simulink model "HyEQ_Optimized"  (Simulink 7.7)
settings: Solver=ode45  StartTime=0.0  StopTime=T  MaxStep=MaxStep  RelTol=RelTol
undefined symbols (not defined in the file or in its folder): J, rule, T, x0
libraries: simulink x6
settings Model: Creator=pablonanez  LastModifiedBy=pablonanez
settings SFSimCC: SimParseCustomCode=off

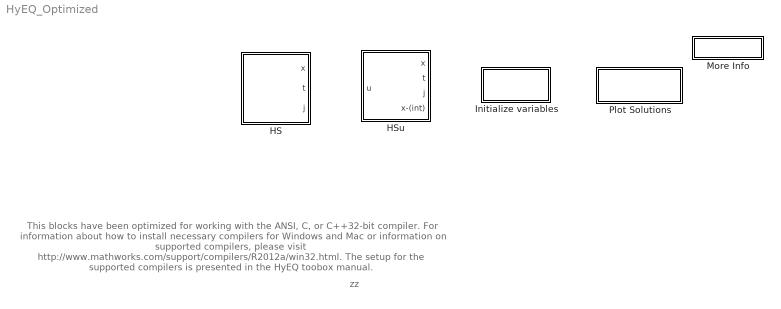
== system HyEQ_Optimized ==
  note: zz
  note: This blocks have been optimized for working with the ANSI, C, or C++32-bit compiler.
      |
      | For information about how to install necessary compilers for Windows and Mac or
      | information on supported compilers, please visit
      | http://www.mathworks.com/support/compilers/R2012a/win32.html.
      |
      | The setup for the supported compilers is presented in the HyEQ toobox manual.
  HS : Subsystem  LoadFcn=set_param(gcb,'LinkStatus','none')
      settings: CopyFcn=|
      | set_param(gcb,'LinkStatus','none'),
      | set_param(gcs, 'MaxStep', 'MaxStep', 'RelTol','RelTol','Stop time', 'T')
      mask Display:
      | image(imread('Hcal.jpg'))
      | %plot([5 20 20 5 5],[5 5 20 20 5])
      | %text(8,13,'HyEq_mdl')
      | port_label('output', 1, 'x')
      | port_label('output', 2, 't')
      | port_label('output', 3, 'j')
  HSu : Subsystem  LoadFcn=set_param(gcb,'LinkStatus','none')
      settings: CopyFcn=|
      | set_param(gcb,'LinkStatus','none'),
      | set_param(gcs, 'MaxStep', 'MaxStep', 'RelTol', 'RelTol','Stop time', 'T')
      mask Display:
      | image(imread('Hcal.jpg'))
      | %plot([5 20 20 5 5],[5 5 20 20 5])
      | %text(8,13,'HyEq_mdl')
      | port_label('output', 1, 'x')
      | port_label('output', 2, 't')
      | port_label('output', 3, 'j')
      | port_label('output', 4, 'x-(int)')
      | port_label('input', 1, 'u')
  Initialize variables : Subsystem  Priority=-10
      settings: OpenFcn=|
      | try
      |      clearvars -except inifile pathfile_in pathfile_pos posfile
      |      cd(pathfile_in);
      |      eval(inifile);
      | catch
      |      [inifile,pathfile_in] = getInitializationfile;
      |      cd(pathfile_in);
      |      inifile = strrep(inifile,'.m','');
      |      eval(inifile);
      | end
      mask Display: disp('Double Click\n to Initialize')
  More Info : Subsystem
      settings: OpenFcn=helpview 'HyEQ_Toolbox_v201.html'
      mask Display: disp('More Info')
  Plot Solutions : Subsystem
      settings: OpenFcn=|
      | try
      |      cd(pathfile_pos);
      |      eval(posfile);
      | catch
      |      [posfile,pathfile_pos] = getInitializationfile;
      |      cd(pathfile_pos);
      |      posfile = strrep(posfile,'.m','');
      |      eval(posfile);
      | end
      mask Display: disp('Double Click to\n Plot Solutions')

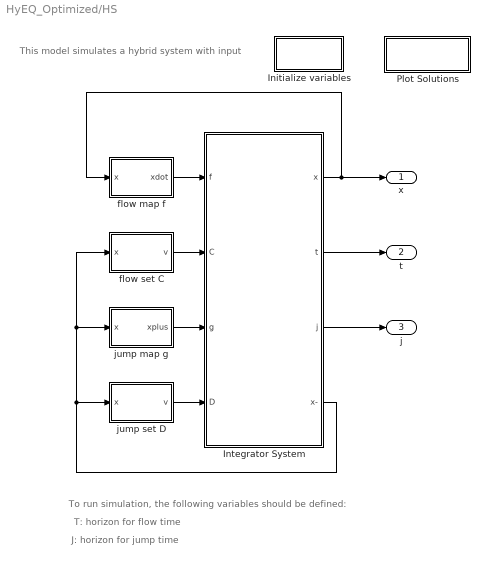
== system HyEQ_Optimized/HS ==
  note: This model simulates a hybrid system with input
  note: To run simulation, the following variables should be defined:
  note: T: horizon for flow time
  note: J: horizon for jump time
  Initialize variables : Subsystem  Priority=-10
      settings: OpenFcn=|
      | try
      |      clearvars -except inifile pathfile_in pathfile_pos posfile
      |      cd(pathfile_in);
      |      eval(inifile);
      | catch
      |      [inifile,pathfile_in] = getInitializationfile;
      |      cd(pathfile_in);
      |      inifile = strrep(inifile,'.m','');
      |      eval(inifile);
      | end
      mask Display: disp('Double Click\n to Initialize')
  Integrator System : Subsystem  Priority=2  mask(Hybrid Integrator){T=T, J=J, x0=x0}
      mask prompts: T "Flow Horizon"; J "Jump Horizon"; x0 "Initial Condition"
      mask help:
      | This block integrates the state of the hybrid system defined by the flow map f (first input), the flow set C (second input), the jump map g (third input) and the jump set D (fourth input).
      | Starting from the initial condition x0 (last mask parameter), the system's state x evolves continuously within the set C, according to f(x,u), but is also subject to jumps within D, according to g(x,u).
      | The block also stops the simulation when the time t is greater than the flow horizon T (first mask parameter), or when the number of jumps j is greater than the jump horizon J (second mask parameter).
      | The outputs of the blocks are respectively x(t), t, j, x(t-).
      mask Help:
      | This block integrates the state of the hybrid system defined by the flow map f (first input), the flow set C (second input), the jump map g (third input) and the jump set D (fourth input).
      | <br>
      | Starting from the initial condition x0 (last mask parameter), the system's state x evolves continuously within the set C, according to f(x,u), but is also subject to jumps within D, according to g(x,u).
      | <br>
      | The block also stops the simulation when the time t is greater than the flow horizon T (first mask parameter), or when the number of jumps j is greater than the jump horizon J (second mask parameter).
      | <br>
      | The outputs of the blocks are respectively x(t), t, j, x(t-).
      | <br>
      | You can right click on the block and "Look under mask" to see what's inside the block.
      | Finally, refer to the manual (HybridSimulator_vXX.pdf) for more detailed information on how this hybrid simulator works.
  Plot Solutions : Subsystem
      settings: OpenFcn=|
      | try
      |      cd(pathfile_pos);
      |      eval(posfile);
      | catch
      |      [posfile,pathfile_pos] = getInitializationfile;
      |      cd(pathfile_pos);
      |      posfile = strrep(posfile,'.m','');
      |      eval(posfile);
      | end
      mask Display: disp('Double Click to\n Plot Solutions')
  flow map f : Stateflow chart  TreatAsAtomicUnit=on
  flow set C : Stateflow chart  TreatAsAtomicUnit=on
  jump map g : Stateflow chart  Priority=2  TreatAsAtomicUnit=on
  jump set D : Stateflow chart  TreatAsAtomicUnit=on
  x : Outport
  t : Outport  Port=2
  j : Outport  Port=3
  wires:
  flow map f/1(xdot) -> Integrator System/1(f)
  Integrator System/4(x-) -> jump map g/1(x), flow set C/1(x), jump set D/1(x)
  Integrator System/1(x) -> flow map f/1(x), x/1
  flow set C/1(v) -> Integrator System/2(C)
  Integrator System/2(t) -> t/1
  Integrator System/3(j) -> j/1
  jump set D/1(v) -> Integrator System/4(D)
  jump map g/1(xplus) -> Integrator System/3(g)

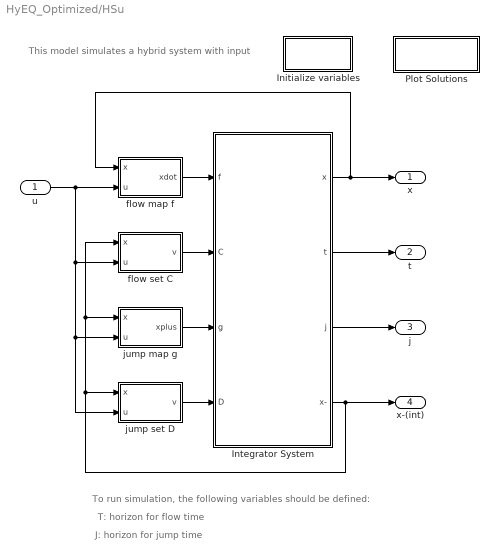
== system HyEQ_Optimized/HSu ==
  note: This model simulates a hybrid system with input
  note: To run simulation, the following variables should be defined:
  note: T: horizon for flow time
  note: J: horizon for jump time
  u : Inport
  Initialize variables : Subsystem  Priority=-10
      settings: OpenFcn=|
      | try
      |      clearvars -except inifile pathfile_in pathfile_pos posfile
      |      cd(pathfile_in);
      |      eval(inifile);
      | catch
      |      [inifile,pathfile_in] = getInitializationfile;
      |      cd(pathfile_in);
      |      inifile = strrep(inifile,'.m','');
      |      eval(inifile);
      | end
      mask Display: disp('Double Click\n to Initialize')
  Integrator System : Subsystem  Priority=2  mask(Hybrid Integrator){T=T, J=J, x0=x0}
      mask prompts: T "Flow Horizon"; J "Jump Horizon"; x0 "Initial Condition"
      mask help:
      | This block integrates the state of the hybrid system defined by the flow map f (first input), the flow set C (second input), the jump map g (third input) and the jump set D (fourth input).
      | Starting from the initial condition x0 (last mask parameter), the system's state x evolves continuously within the set C, according to f(x,u), but is also subject to jumps within D, according to g(x,u).
      | The block also stops the simulation when the time t is greater than the flow horizon T (first mask parameter), or when the number of jumps j is greater than the jump horizon J (second mask parameter).
      | The outputs of the blocks are respectively x(t), t, j, x(t-).
      mask Help:
      | This block integrates the state of the hybrid system defined by the flow map f (first input), the flow set C (second input), the jump map g (third input) and the jump set D (fourth input).
      | <br>
      | Starting from the initial condition x0 (last mask parameter), the system's state x evolves continuously within the set C, according to f(x,u), but is also subject to jumps within D, according to g(x,u).
      | <br>
      | The block also stops the simulation when the time t is greater than the flow horizon T (first mask parameter), or when the number of jumps j is greater than the jump horizon J (second mask parameter).
      | <br>
      | The outputs of the blocks are respectively x(t), t, j, x(t-).
      | <br>
      | You can right click on the block and "Look under mask" to see what's inside the block.
      | Finally, refer to the manual (HybridSimulator_vXX.pdf) for more detailed information on how this hybrid simulator works.
  Plot Solutions : Subsystem
      settings: OpenFcn=|
      | try
      |      cd(pathfile_pos);
      |      eval(posfile);
      | catch
      |      [posfile,pathfile_pos] = getInitializationfile;
      |      cd(pathfile_pos);
      |      posfile = strrep(posfile,'.m','');
      |      eval(posfile);
      | end
      mask Display: disp('Double Click to\n Plot Solutions')
  flow map f : Stateflow chart  TreatAsAtomicUnit=on
  flow set C : Stateflow chart  TreatAsAtomicUnit=on
  jump map g : Stateflow chart  Priority=2  TreatAsAtomicUnit=on
  jump set D : Stateflow chart  TreatAsAtomicUnit=on
  x : Outport
  t : Outport  Port=2
  j : Outport  Port=3
  x-(int) : Outport  Port=4
  wires:
  flow map f/1(xdot) -> Integrator System/1(f)
  Integrator System/4(x-) -> jump map g/1(x), flow set C/1(x), jump set D/1(x), x-(int)/1
  Integrator System/1(x) -> flow map f/1(x), x/1
  flow set C/1(v) -> Integrator System/2(C)
  Integrator System/2(t) -> t/1
  Integrator System/3(j) -> j/1
  u/1 -> flow map f/2(u), flow set C/2(u), jump map g/2(u), jump set D/2(u)
  jump set D/1(v) -> Integrator System/4(D)
  jump map g/1(xplus) -> Integrator System/3(g)

== system HyEQ_Optimized/Initialize variables ==

== system HyEQ_Optimized/More Info ==

== system HyEQ_Optimized/Plot Solutions ==

== system HyEQ_Optimized/HS/Initialize variables ==

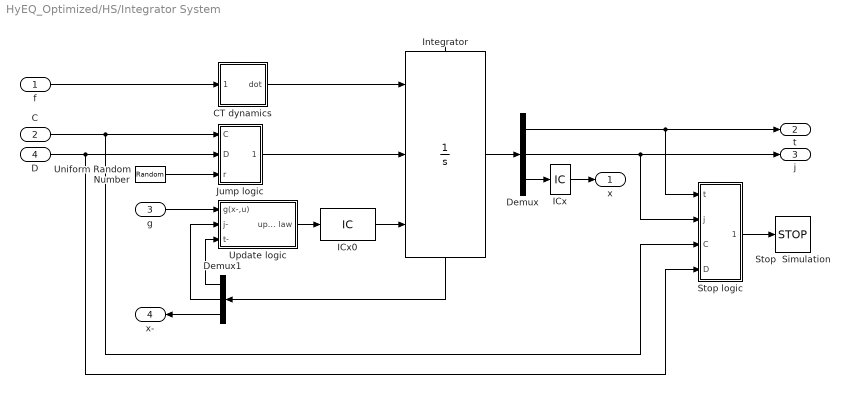
== system HyEQ_Optimized/HS/Integrator System ==
  f : Inport
  C : Inport  Port=2
  g : Inport  Port=3
  D : Inport  Port=4
  CT dynamics : Subsystem
  Demux : Demux  Outputs=[1 1 -1]
  Demux1 : Demux  Outputs=[1 1 -1]
  ICx : InitialCondition  Value=x0
  ICx0 : InitialCondition  Value=[0; 0; x0(:)]
  Integrator : Integrator  ExternalReset=level hold  InitialConditionSource=external  ShowStatePort=on  ZeroCross=off
  Jump logic : Subsystem
  Stop  Simulation : Stop
  Stop logic : Subsystem
  Uniform Random Number : UniformRandomNumber  Minimum=0  Seed=abs(floor(100*rand))  SampleTime=0
  Update logic : Subsystem
  x : Outport
  t : Outport  Port=2
  j : Outport  Port=3
  x- : Outport  Port=4
  wires:
  Demux1/2 -> Update logic/2(j-)
  Demux1/1 -> Update logic/3(t-)
  g/1 -> Update logic/1(g(x-,u))
  Uniform Random Number/1 -> Jump logic/3(r)
  Jump logic/1(jump) -> Integrator/2
  Demux1/3 -> x-/1
  f/1 -> CT dynamics/1(f(x,u))
  D/1 -> Jump logic/2(D), Stop logic/4(D)
  C/1 -> Jump logic/1(C), Stop logic/3(C)
  Integrator/1 -> Demux/1
  Stop logic/1(stop) -> Stop  Simulation/1
  CT dynamics/1(dot) -> Integrator/1
  Update logic/1(update law) -> ICx0/1
  Demux/1 -> Stop logic/1(t), t/1
  Demux/2 -> Stop logic/2(j), j/1
  Integrator/State -> Demux1/1
  Demux/3 -> ICx/1
  ICx/1 -> x/1
  ICx0/1 -> Integrator/3

== system HyEQ_Optimized/HS/Plot Solutions ==

== system HyEQ_Optimized/HSu/Initialize variables ==

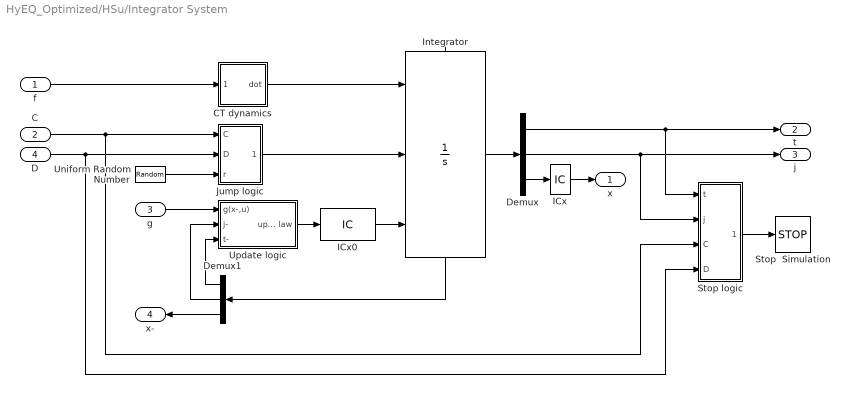
== system HyEQ_Optimized/HSu/Integrator System ==
  f : Inport
  C : Inport  Port=2
  g : Inport  Port=3
  D : Inport  Port=4
  CT dynamics : Subsystem
  Demux : Demux  Outputs=[1 1 -1]
  Demux1 : Demux  Outputs=[1 1 -1]
  ICx : InitialCondition  Value=x0
  ICx0 : InitialCondition  Value=[0; 0; x0(:)]
  Integrator : Integrator  ExternalReset=level hold  InitialConditionSource=external  ShowStatePort=on  ZeroCross=off
  Jump logic : Subsystem
  Stop  Simulation : Stop
  Stop logic : Subsystem
  Uniform Random Number : UniformRandomNumber  Minimum=0  Seed=abs(floor(100*rand))  SampleTime=0
  Update logic : Subsystem
  x : Outport
  t : Outport  Port=2
  j : Outport  Port=3
  x- : Outport  Port=4
  wires:
  Demux1/2 -> Update logic/2(j-)
  Demux1/1 -> Update logic/3(t-)
  g/1 -> Update logic/1(g(x-,u))
  Uniform Random Number/1 -> Jump logic/3(r)
  Jump logic/1(jump) -> Integrator/2
  Demux1/3 -> x-/1
  f/1 -> CT dynamics/1(f(x,u))
  D/1 -> Jump logic/2(D), Stop logic/4(D)
  C/1 -> Jump logic/1(C), Stop logic/3(C)
  Integrator/1 -> Demux/1
  Stop logic/1(stop) -> Stop  Simulation/1
  CT dynamics/1(dot) -> Integrator/1
  Update logic/1(update law) -> ICx0/1
  Demux/1 -> Stop logic/1(t), t/1
  Demux/2 -> Stop logic/2(j), j/1
  Integrator/State -> Demux1/1
  Demux/3 -> ICx/1
  ICx/1 -> x/1
  ICx0/1 -> Integrator/3

== system HyEQ_Optimized/HSu/Plot Solutions ==

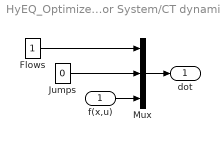
== system HyEQ_Optimized/HS/Integrator System/CT dynamics ==
  f(x,u) : Inport
  Flows : Constant
  Jumps : Constant  Value=0
  Mux : Mux  Inputs=[1 1 -1]
  dot : Outport
  wires:
  f(x,u)/1 -> Mux/3
  Mux/1 -> dot/1
  Flows/1 -> Mux/1
  Jumps/1 -> Mux/2

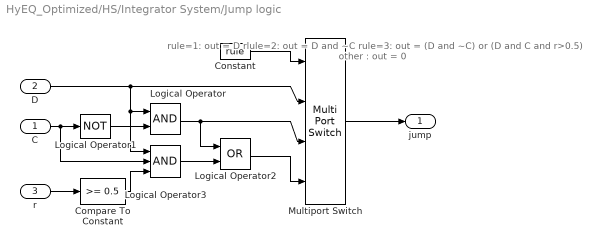
== system HyEQ_Optimized/HS/Integrator System/Jump logic ==
  note: rule=1:  out = D
      | rlule=2: out = D and ~C
      | rule=3:  out = (D and ~C)  or (D and C and r>0.5)
      | other :  out = 0
  C : Inport
  D : Inport  Port=2
  r : Inport  Port=3
  Compare To Constant : simulink/Logic and Bit Operations/Compare To Constant  SystemSampleTime=-1  relop=>=  const=0.5  LogicOutDataTypeMode=uint8
  Constant : Constant  Value=rule
  Logical Operator : Logic  AllPortsSameDT=off  OutDataTypeStr=boolean
  Logical Operator1 : Logic  Operator=NOT  Inputs=1  AllPortsSameDT=off  OutDataTypeStr=boolean
  Logical Operator2 : Logic  Operator=OR  AllPortsSameDT=off  OutDataTypeStr=boolean
  Logical Operator3 : Logic  Inputs=3  AllPortsSameDT=off  OutDataTypeStr=boolean
  Multiport Switch : MultiPortSwitch  zeroidx=off
  jump : Outport
  wires:
  Logical Operator3/1 -> Logical Operator2/2
  Compare To Constant/1 -> Logical Operator3/3
  Multiport Switch/1 -> jump/1
  Logical Operator2/1 -> Multiport Switch/4
  Logical Operator/1 -> Logical Operator2/1, Multiport Switch/3
  Logical Operator1/1 -> Logical Operator/2
  C/1 -> Logical Operator1/1, Logical Operator3/2
  r/1 -> Compare To Constant/1
  D/1 -> Multiport Switch/2, Logical Operator/1, Logical Operator3/1
  Constant/1 -> Multiport Switch/1

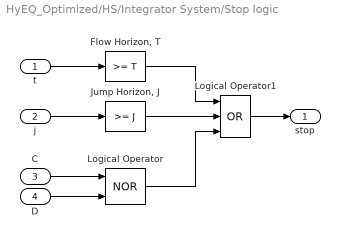
== system HyEQ_Optimized/HS/Integrator System/Stop logic ==
  t : Inport
  j : Inport  Port=2
  C : Inport  Port=3
  D : Inport  Port=4
  "Flow Horizon, T" : simulink/Logic and Bit Operations/Compare To Constant  SystemSampleTime=-1  relop=>=  const=T  LogicOutDataTypeMode=uint8  ZeroCross=off
  "Jump Horizon, J" : simulink/Logic and Bit Operations/Compare To Constant  SystemSampleTime=-1  relop=>=  const=J  LogicOutDataTypeMode=uint8  ZeroCross=off
  Logical Operator : Logic  Operator=NOR  AllPortsSameDT=off  OutDataTypeStr=boolean
  Logical Operator1 : Logic  Operator=OR  Inputs=3  AllPortsSameDT=off  OutDataTypeStr=boolean
  stop : Outport
  wires:
  Logical Operator1/1 -> stop/1
  C/1 -> Logical Operator/1
  j/1 -> "Jump Horizon, J"/1
  t/1 -> "Flow Horizon, T"/1
  D/1 -> Logical Operator/2
  Logical Operator/1 -> Logical Operator1/3
  "Jump Horizon, J"/1 -> Logical Operator1/2
  "Flow Horizon, T"/1 -> Logical Operator1/1

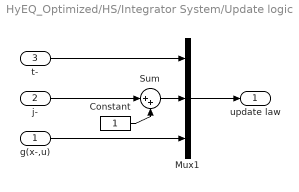
== system HyEQ_Optimized/HS/Integrator System/Update logic ==
  g(x-,u) : Inport
  j- : Inport  Port=2
  t- : Inport  Port=3
  Constant : Constant
  Mux1 : Mux  Inputs=[1 1 -1]
  Sum : Sum  Inputs=|++
  update law : Outport
  wires:
  Constant/1 -> Sum/2
  t-/1 -> Mux1/1
  g(x-,u)/1 -> Mux1/3
  j-/1 -> Sum/1
  Mux1/1 -> update law/1
  Sum/1 -> Mux1/2

== system HyEQ_Optimized/HSu/Integrator System/CT dynamics ==
  f(x,u) : Inport
  Flows : Constant
  Jumps : Constant  Value=0
  Mux : Mux  Inputs=[1 1 -1]
  dot : Outport
  wires:
  f(x,u)/1 -> Mux/3
  Mux/1 -> dot/1
  Flows/1 -> Mux/1
  Jumps/1 -> Mux/2

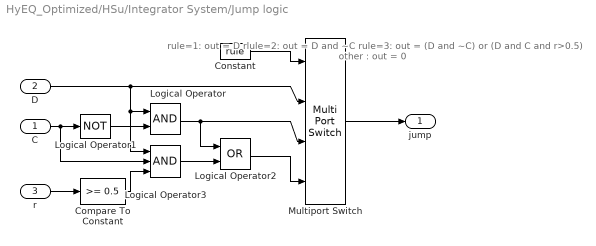
== system HyEQ_Optimized/HSu/Integrator System/Jump logic ==
  note: rule=1:  out = D
      | rlule=2: out = D and ~C
      | rule=3:  out = (D and ~C)  or (D and C and r>0.5)
      | other :  out = 0
  C : Inport
  D : Inport  Port=2
  r : Inport  Port=3
  Compare To Constant : simulink/Logic and Bit Operations/Compare To Constant  SystemSampleTime=-1  relop=>=  const=0.5  LogicOutDataTypeMode=uint8
  Constant : Constant  Value=rule
  Logical Operator : Logic  AllPortsSameDT=off  OutDataTypeStr=boolean
  Logical Operator1 : Logic  Operator=NOT  Inputs=1  AllPortsSameDT=off  OutDataTypeStr=boolean
  Logical Operator2 : Logic  Operator=OR  AllPortsSameDT=off  OutDataTypeStr=boolean
  Logical Operator3 : Logic  Inputs=3  AllPortsSameDT=off  OutDataTypeStr=boolean
  Multiport Switch : MultiPortSwitch  zeroidx=off
  jump : Outport
  wires:
  Logical Operator3/1 -> Logical Operator2/2
  Compare To Constant/1 -> Logical Operator3/3
  Multiport Switch/1 -> jump/1
  Logical Operator2/1 -> Multiport Switch/4
  Logical Operator/1 -> Logical Operator2/1, Multiport Switch/3
  Logical Operator1/1 -> Logical Operator/2
  C/1 -> Logical Operator1/1, Logical Operator3/2
  r/1 -> Compare To Constant/1
  D/1 -> Multiport Switch/2, Logical Operator/1, Logical Operator3/1
  Constant/1 -> Multiport Switch/1

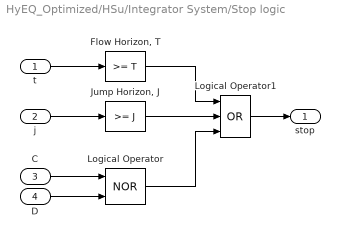
== system HyEQ_Optimized/HSu/Integrator System/Stop logic ==
  t : Inport
  j : Inport  Port=2
  C : Inport  Port=3
  D : Inport  Port=4
  "Flow Horizon, T" : simulink/Logic and Bit Operations/Compare To Constant  SystemSampleTime=-1  relop=>=  const=T  LogicOutDataTypeMode=uint8  ZeroCross=off
  "Jump Horizon, J" : simulink/Logic and Bit Operations/Compare To Constant  SystemSampleTime=-1  relop=>=  const=J  LogicOutDataTypeMode=uint8  ZeroCross=off
  Logical Operator : Logic  Operator=NOR  AllPortsSameDT=off  OutDataTypeStr=boolean
  Logical Operator1 : Logic  Operator=OR  Inputs=3  AllPortsSameDT=off  OutDataTypeStr=boolean
  stop : Outport
  wires:
  Logical Operator1/1 -> stop/1
  C/1 -> Logical Operator/1
  j/1 -> "Jump Horizon, J"/1
  t/1 -> "Flow Horizon, T"/1
  D/1 -> Logical Operator/2
  Logical Operator/1 -> Logical Operator1/3
  "Jump Horizon, J"/1 -> Logical Operator1/2
  "Flow Horizon, T"/1 -> Logical Operator1/1

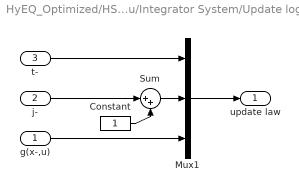
== system HyEQ_Optimized/HSu/Integrator System/Update logic ==
  g(x-,u) : Inport
  j- : Inport  Port=2
  t- : Inport  Port=3
  Constant : Constant
  Mux1 : Mux  Inputs=[1 1 -1]
  Sum : Sum  Inputs=|++
  update law : Outport
  wires:
  Constant/1 -> Sum/2
  t-/1 -> Mux1/1
  g(x-,u)/1 -> Mux1/3
  j-/1 -> Sum/1
  Mux1/1 -> update law/1
  Sum/1 -> Mux1/2

== matlab function HSu/jump set D ==
  data: x input double; v output double; u input double
function v  = D(x, u) 
%--------------------------------------------------------------------------
% Matlab M-file Project: HyEQ Toolbox @  Hybrid Systems Laboratory (HSL), 
% https://hybrid.soe.ucsc.edu/software
% http://hybridsimulator.wordpress.com/
%--------------------------------------------------------------------------
% Project: Simulation of a hybrid system
% Description: Jump set
%--------------------------------------------------------------------------
%--------------------------------------------------------------------------
%   See also plotflows, plotHarc, plotHarcColor, plotHarcColor3D,
%   plotHybridArc, plotjumps.
%   Copyright @ Hybrid Systems Laboratory (HSL),
%   Revision: 0.0.0.3 Date: 05/20/2015 3:42:00
%
% Check on jump conditions
% % E.g.,
% if (x(1) <= u(1)) && (x(2) <= 0)  % jump condition
%     v = 1;  % report jump
% else
%     v = 0;   % do not report jump
% end

v = 0;

== matlab function HSu/flow map f ==
  data: x input double; xdot output double; u input double
function xdot = f(x, u)
%--------------------------------------------------------------------------
% Matlab M-file Project: HyEQ Toolbox @  Hybrid Systems Laboratory (HSL), 
% https://hybrid.soe.ucsc.edu/software
% http://hybridsimulator.wordpress.com/
%--------------------------------------------------------------------------
% Project: Simulation of a hybrid system
% Description: Flow map
%--------------------------------------------------------------------------
%--------------------------------------------------------------------------
%   See also plotflows, plotHarc, plotHarcColor, plotHarcColor3D,
%   plotHybridArc, plotjumps.
%   Copyright @ Hybrid Systems Laboratory (HSL),
%   Revision: 0.0.0.3 Date: 05/20/2015 3:42:00
%--------------------------------------------------------------------------
% flow map: xdot=f(x,u);

xdot = 0;

== matlab function HS/flow map f ==
  data: x input double; xdot output double
function xdot = f(x)
%--------------------------------------------------------------------------
% Matlab M-file Project: HyEQ Toolbox @  Hybrid Systems Laboratory (HSL), 
% https://hybrid.soe.ucsc.edu/software
% http://hybridsimulator.wordpress.com/
%--------------------------------------------------------------------------
% Project: Simulation of a hybrid system
% Description: Flow map
%--------------------------------------------------------------------------
%--------------------------------------------------------------------------
%   See also plotflows, plotHarc, plotHarcColor, plotHarcColor3D,
%   plotHybridArc, plotjumps.
%   Copyright @ Hybrid Systems Laboratory (HSL),
%   Revision: 0.0.0.3 Date: 05/20/2015 3:42:00

xdot = 0;

== matlab function HS/flow set C ==
  data: x input double; v output double
function v  = C(x) 
%--------------------------------------------------------------------------
% Matlab M-file Project: HyEQ Toolbox @  Hybrid Systems Laboratory (HSL), 
% https://hybrid.soe.ucsc.edu/software
% http://hybridsimulator.wordpress.com/
%--------------------------------------------------------------------------
% Project: Simulation of a hybrid system
% Description: Flow set
%--------------------------------------------------------------------------
%--------------------------------------------------------------------------
%   See also plotflows, plotHarc, plotHarcColor, plotHarcColor3D,
%   plotHybridArc, plotjumps.
%   Copyright @ Hybrid Systems Laboratory (HSL),
%   Revision: 0.0.0.3 Date: 05/20/2015 3:42:00
%
% Check on flow conditions
% E.g.,
% if (x(1) >= u(1))  % flow condition
%     v = 1;  % report flow
% else
%     v = 0;   % do not report flow
% end

v = 0;

== matlab function HS/jump map g ==
  data: x input double; xplus output double
function xplus = g(x)
%--------------------------------------------------------------------------
% Matlab M-file Project: HyEQ Toolbox @  Hybrid Systems Laboratory (HSL), 
% https://hybrid.soe.ucsc.edu/software
% http://hybridsimulator.wordpress.com/
%--------------------------------------------------------------------------
% Project: Simulation of a hybrid system
% Description: Jump map
%--------------------------------------------------------------------------
%--------------------------------------------------------------------------
%   See also plotflows, plotHarc, plotHarcColor, plotHarcColor3D,
%   plotHybridArc, plotjumps.
%   Copyright @ Hybrid Systems Laboratory (HSL),
%   Revision: 0.0.0.3 Date: 05/20/2015 3:42:00

xplus = 0;

== matlab function HSu/flow set C ==
  data: x input double; v output double; u input double
function v  = C(x, u) 
%--------------------------------------------------------------------------
% Matlab M-file Project: HyEQ Toolbox @  Hybrid Systems Laboratory (HSL), 
% https://hybrid.soe.ucsc.edu/software
% http://hybridsimulator.wordpress.com/
%--------------------------------------------------------------------------
% Project: Simulation of a hybrid system
% Description: Flow set
%--------------------------------------------------------------------------
%--------------------------------------------------------------------------
%   See also plotflows, plotHarc, plotHarcColor, plotHarcColor3D,
%   plotHybridArc, plotjumps.
%   Copyright @ Hybrid Systems Laboratory (HSL),
%   Revision: 0.0.0.3 Date: 05/20/2015 3:42:00
%
% Check on flow conditions
% E.g.,
% if (x(1) >= u(1))  % flow condition
%     v = 1;  % report flow
% else
%     v = 0;   % do not report flow
% end

v = 0;

== matlab function HSu/jump map g ==
  data: x input double; xplus output double; u input double
function xplus = g(x, u)
%--------------------------------------------------------------------------
% Matlab M-file Project: HyEQ Toolbox @  Hybrid Systems Laboratory (HSL), 
% https://hybrid.soe.ucsc.edu/software
% http://hybridsimulator.wordpress.com/
%--------------------------------------------------------------------------
% Project: Simulation of a hybrid system
% Description: Jump map
%--------------------------------------------------------------------------
%--------------------------------------------------------------------------
%   See also plotflows, plotHarc, plotHarcColor, plotHarcColor3D,
%   plotHybridArc, plotjumps.
%   Copyright @ Hybrid Systems Laboratory (HSL),
%   Revision: 0.0.0.3 Date: 05/20/2015 3:42:00
%--------------------------------------------------------------------------
% jump map: xplus = g(x,u);

xplus = 0;

== matlab function HS/jump set D ==
  data: x input double; v output double
function v  = D(x) 
%--------------------------------------------------------------------------
% Matlab M-file Project: HyEQ Toolbox @  Hybrid Systems Laboratory (HSL), 
% https://hybrid.soe.ucsc.edu/software
% http://hybridsimulator.wordpress.com/
%--------------------------------------------------------------------------
% Project: Simulation of a hybrid system
% Description: Jump set
%--------------------------------------------------------------------------
%--------------------------------------------------------------------------
%   See also plotflows, plotHarc, plotHarcColor, plotHarcColor3D,
%   plotHybridArc, plotjumps.
%   Copyright @ Hybrid Systems Laboratory (HSL),
%   Revision: 0.0.0.3 Date: 05/20/2015 3:42:00
%
% Check on jump conditions
% % E.g.,
% if (x(1) <= u(1)) && (x(2) <= 0)  % jump condition
%     v = 1;  % report jump
% else
%     v = 0;   % do not report jump
% end

v = 0;
